simulink model "battery_PV_microgrid"  (R2014a)
settings: Solver=ode23tb  StartTime=0.0  StopTime=86000  MaxStep=0.2  RelTol=1e-5
InitFcn:
  | % Load Stateflow/Controller Parameters
  | controlParams();
  | 
  | % Load Initial Conditions for Model
  | initialConditions();
  | 
  | % Load Battery/PV Parameters
  | parameters();
StopFcn:
  | % Plot results
  | %plotSimResults();
values from neighbouring files (symbols this model uses):
  ambientTemp = 20    [initialConditions.m]    (also in initializeBattery.m)
  currentSat = 0.5    [controlParams.m]    (also in initializeBattery.m)
  desiredBusVoltage = 30    [controlParams.m]    (also in initializeBattery.m = 24.45)
  finalVoltage = 30    [controlParams.m]    (also in initializeBattery.m = 26)
  maxChargeRate = 5    [controlParams.m]    (also in initializeBattery.m)
  maxDischargeRate = -5    [controlParams.m]    (also in initializeBattery.m)
  Ncell = 100    [parameters.m]
  T_init = ambientTemp + 273.15    (= 293.15)    [initialConditions.m]    (also in initializeBattery.m)
  tau = 1e-4    (= 0.0001)    [parameters.m]
undefined symbols (not defined in the file or in its folder): hysteresisSOC, Ion, Lithium, maxSOC, minSOC, optTime, powerHysteresis
undefined symbols (not defined in the file): C1_LUT, C2_LUT, Capacity_LUT, cell_Cp_heat, cell_mass, Em_LUT, PVCellIsc, PVCellRs, PVCellVoc, Qe_init, R0_LUT, R1_LUT, R2_LUT, SOC_LUT, Temperature_LUT
libraries: powerlib x49, fl_lib x18, nesl_utility x6, LiBatteryElements_lib x6, simulink x3, simulink_extras x3, electricdrivelib x1
(part 2 of 2)

== system battery_PV_microgrid/Battery//PV Management and Control/Battery Charge//Discharge Controllers/Battery Charge Controller ==
  Controller Mode : Inport
  Measurements : Inport  Port=2
  Action Port : ActionPort  InitializeStates=reset  ActionType=case
  Bus Selector : BusSelector  OutputSignals=bus.BattVoltage,bus.BattCurrent
  Constant Charge Current : Constant  Value=maxChargeRate
  Final Cell Voltage : Constant  Value=finalVoltage
  Multiport Switch : MultiPortSwitch  DataPortOrder=Zero-based contiguous  Inputs=2
  PID Controller : simulink/Continuous/PID Controller  Controller=PID  TimeDomain=Continuous-time  SampleTime=-1  IntegratorMethod=Forward Euler  FilterMethod=Forward Euler  Form=Parallel  P=1  I=1  D=0.1  N=100  InitialConditionSource=internal  InitialConditionForIntegrator=0  InitialConditionForFilter=0  ExternalReset=none  LimitOutput=on  UpperSaturationLimit=1  LowerSaturationLimit=0  LinearizeAsGain=on  AntiWindupMode=back-calculation  Kb=1  TrackingMode=off  Kt=1  PParamMin=[]  PParamMax=[]  IParamMin=[]  IParamMax=[]  DParamMin=[]  DParamMax=[]  NParamMin=[]  NParamMax=[]  KbParamMin=[]  KbParamMax=[]  KtParamMin=[]  KtParamMax=[]  POutMin=[]  POutMax=[]  IOutMin=[]  IOutMax=[]  DOutMin=[]  DOutMax=[]  NOutMin=[]  NOutMax=[]  KbOutMin=[]  KbOutMax=[]  KtOutMin=[]  KtOutMax=[]  IntegratorOutMin=[]  IntegratorOutMax=[]  FilterOutMin=[]  FilterOutMax=[]  SumOutMin=[]  SumOutMax=[]  SumI1OutMin=[]  SumI1OutMax=[]  SumI2OutMin=[]  SumI2OutMax=[]  SumI3OutMin=[]  SumI3OutMax=[]  SumDOutMin=[]  SumDOutMax=[]  SaturationOutMin=[]  SaturationOutMax=[]  IntegratorContinuousStateAttributes=''  IntegratorStateMustResolveToSignalObject=off  IntegratorRTWStateStorageClass=Auto  FilterContinuousStateAttributes=''  FilterStateMustResolveToSignalObject=off  FilterRTWStateStorageClass=Auto
  Selected Mode : Scope
      settings: ShowLegends=on  TimeRange=4000  YMin=-100  YMax=1400  SaveName=mode
  Sum : Sum  Inputs=|+-
  Sum1 : Sum  Inputs=|+-
  scaling : Subsystem
  Duty : Outport
  wires:
  Multiport Switch/1 -> PID Controller/1
  Constant Charge Current/1 -> Sum/1
  Final Cell Voltage/1 -> Sum1/1
  Sum1/1 -> Multiport Switch/2
  Sum/1 -> Multiport Switch/3
  scaling/1(m) -> Duty/1
  PID Controller/1 -> scaling/1(D)
  Controller Mode/1 -> Selected Mode/1, Multiport Switch/1
  Measurements/1 -> Bus Selector/1
  Bus Selector/1 -> Sum1/2  "<BattVoltage>"
  Bus Selector/2 -> Sum/2  "<BattCurrent>"

== system battery_PV_microgrid/Battery//PV Management and Control/Battery Charge//Discharge Controllers/Battery Discharge Controller ==
  Controller Mode : Inport
  Measurements : Inport  Port=2
  Action Port : ActionPort  InitializeStates=reset  ActionType=default
  Bus Selector : BusSelector  OutputSignals=bus.BattCurrent,bus.BusVoltage
  Maximum Desired Current Output : Constant  Value=maxDischargeRate
  Maximum Desired Current Output1 : Constant  Value=desiredBusVoltage
  Multiport Switch : MultiPortSwitch  DataPortOrder=Zero-based contiguous  Inputs=2
  PID Controller : simulink/Continuous/PID Controller  Controller=PID  TimeDomain=Continuous-time  SampleTime=-1  IntegratorMethod=Forward Euler  FilterMethod=Forward Euler  Form=Parallel  P=1  I=10  D=0  N=100  InitialConditionSource=internal  InitialConditionForIntegrator=0  InitialConditionForFilter=0  ExternalReset=none  LimitOutput=on  UpperSaturationLimit=1  LowerSaturationLimit=0  LinearizeAsGain=on  AntiWindupMode=back-calculation  Kb=1  TrackingMode=off  Kt=1  PParamMin=[]  PParamMax=[]  IParamMin=[]  IParamMax=[]  DParamMin=[]  DParamMax=[]  NParamMin=[]  NParamMax=[]  KbParamMin=[]  KbParamMax=[]  KtParamMin=[]  KtParamMax=[]  POutMin=[]  POutMax=[]  IOutMin=[]  IOutMax=[]  DOutMin=[]  DOutMax=[]  NOutMin=[]  NOutMax=[]  KbOutMin=[]  KbOutMax=[]  KtOutMin=[]  KtOutMax=[]  IntegratorOutMin=[]  IntegratorOutMax=[]  FilterOutMin=[]  FilterOutMax=[]  SumOutMin=[]  SumOutMax=[]  SumI1OutMin=[]  SumI1OutMax=[]  SumI2OutMin=[]  SumI2OutMax=[]  SumI3OutMin=[]  SumI3OutMax=[]  SumDOutMin=[]  SumDOutMax=[]  SaturationOutMin=[]  SaturationOutMax=[]  IntegratorContinuousStateAttributes=''  IntegratorStateMustResolveToSignalObject=off  IntegratorRTWStateStorageClass=Auto  FilterContinuousStateAttributes=''  FilterStateMustResolveToSignalObject=off  FilterRTWStateStorageClass=Auto
  Selected Mode : Scope
      settings: YMin=0.95  YMax=1.05  SaveName=mode2
  Selected Mode1 : Scope
      settings: YMin=0.95  YMax=1.05  SaveName=mode1
  Sum : Sum  Inputs=|+-
  Sum1 : Sum  Inputs=|-+
  scaling : Subsystem
  Duty : Outport
  wires:
  scaling/1(m) -> Duty/1
  Maximum Desired Current Output/1 -> Sum1/1
  Bus Selector/1 -> Sum1/2  "<BattCurrent>"
  Multiport Switch/1 -> Selected Mode1/1, PID Controller/1
  PID Controller/1 -> scaling/1(D)
  Sum1/1 -> Multiport Switch/2
  Sum/1 -> Multiport Switch/3
  Bus Selector/2 -> Sum/2  "<BusVoltage>"
  Controller Mode/1 -> Selected Mode/1, Multiport Switch/1
  Measurements/1 -> Bus Selector/1
  Maximum Desired Current Output1/1 -> Sum/1

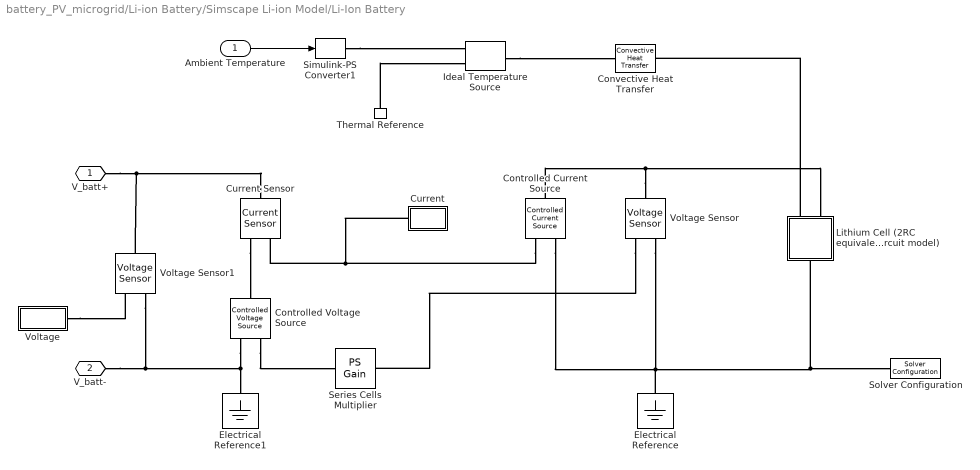
== system battery_PV_microgrid/Li-ion Battery/Simscape Li-ion Model/Li-Ion Battery ==
  Ambient Temperature : Inport
  Controlled Current Source : fl_lib/Electrical/Electrical Sources/Controlled Current Source
  Controlled Voltage Source : fl_lib/Electrical/Electrical Sources/Controlled Voltage Source
  Convective Heat Transfer : fl_lib/Thermal/Thermal Elements/Convective Heat Transfer  area=cell_area m^2  heat_tr_coeff=h_conv W/(m^2 * K)  Q_specify=off  Q_priority=High  Q=0 J/s  T_specify=off  T_priority=High  T=0 K
  Current : Subsystem
  Current Sensor : fl_lib/Electrical/Electrical Sensors/Current Sensor
  Electrical Reference : fl_lib/Electrical/Electrical Elements/Electrical Reference
  Electrical Reference1 : fl_lib/Electrical/Electrical Elements/Electrical Reference
  Ideal Temperature Source : fl_lib/Thermal/Thermal Sources/Ideal Temperature Source
  Lithium Cell (2RC equivalent circuit model) : Subsystem  mask(Lithium battery (two RC-branch equivalent circuit)){Qe_init=Qe_init, T_init=T_init, Capacity_LUT=Capacity_LUT, Em_LUT=Em_LUT, R0_LUT=R0_LUT, R1_LUT=R1_LUT, C1_LUT=C1_LUT, R2_LUT=R2_LUT, C2_LUT=C2_LUT, cell_mass=cell_mass, cell_Cp_heat=cell_Cp_heat, SOC_LUT=SOC_LUT, Temperature_LUT=Temperature_LUT}
      mask prompts: Qe_init "Initial charge deficit (A*hr)"; T_init "Initial cell temperature (K)"; Capacity_LUT "Capacity (A*hr, 1xN table)"; Em_LUT "Em open-circuit voltage (volts, MxN table)"; R0_LUT "R0 terminal resistance (ohms, MxN table)"; R1_LUT "R1 resistance (ohms, MxN table)"; C1_LUT "C1 capacitance (farads, MxN table)"; R2_LUT "R2 resistance (ohms, MxN table)"; C2_LUT "C2 capacitance (farads, MxN table)"; cell_mass "Cell mass (kg)"; cell_Cp_heat "Cell specific heat (J/kg/K)"; SOC_LUT "SOC table breakpoints (Mx1 array)"; Temperature_LUT "Temperature table breakpoints(K, 1xN array)"
      mask Display:
      | image(imread('battery.jpg'))
      | color('red')
      | port_label('LConn',1,'H')
      | port_label('LConn',2,'+')
      | port_label('RConn',1,'-')
  Series Cells Multiplier : fl_lib/Physical Signals/Functions/PS Gain  gain=7
  Simulink-PS Converter1 : nesl_utility/Simulink-PS Converter  PhysicalDomain=network_engine_domain  SubClassName=ps_input  LeftPortType=input  RightPortType=output  PseudoPeriodic=off  Frequencies=[]  NoiseDistribution=none  NoiseParameters=[]  Unit=C  AffineConversion=on  InputFiltering=off  SimscapeFilterOrder=1  InputFilterTimeConstant=.001  UdotUserProvided=1
  Solver Configuration : nesl_utility/Solver Configuration  PhysicalDomain=network_engine_domain  SubClassName=solver  LeftPortType=input  RightPortType=generic  Accelerate=off  Tones=[]  Harmonics=[]  SimulateNoise=off  Profile=off  UseLocalSampling=off  EnableSwitchedLinearOptims=on  FrequencyDomain=off  UseCCode=off  RelTol=0.001  AbsTol=1e-06  MinStep=1e-09  ToWorkspace=off  DoDC=on  ResidualTolerance=1e-9  UseLocalSolver=off  LocalSolverChoice=NE_BACKWARD_EULER_ADVANCER  LocalSolverSampleTime=1  DoFixedCost=off  MaxNonlinIter=3  MaxModeIter=2  LinearAlgebra=Sparse  DelaysMemoryBudget=1024  AutomaticFiltering=on  FilteringTimeConstant=0.001
  Thermal Reference : fl_lib/Thermal/Thermal Elements/Thermal Reference
  Voltage : Subsystem
  Voltage Sensor : fl_lib/Electrical/Electrical Sensors/Voltage Sensor
  Voltage Sensor1 : fl_lib/Electrical/Electrical Sensors/Voltage Sensor
  V_batt+ : PMIOPort  Port=1  Side=Left
  V_batt- : PMIOPort  Port=2  Side=Left
  wires:
  Ambient Temperature/1 -> Simulink-PS Converter1/1
  connections:
  V_batt+/RConn1 -- Voltage Sensor1/LConn1 -- Current Sensor/LConn1
  Controlled Voltage Source/RConn2 -- Voltage Sensor1/RConn2 -- V_batt-/RConn1 -- Electrical Reference1/LConn1
  Lithium Cell (2RC equivalent circuit model)/LConn1 -- Convective Heat Transfer/RConn1
  Thermal Reference/LConn1 -- Ideal Temperature Source/RConn2
  Simulink-PS Converter1/RConn1 -- Ideal Temperature Source/RConn1
  Ideal Temperature Source/LConn1 -- Convective Heat Transfer/LConn1
  Electrical Reference/LConn1 -- Lithium Cell (2RC equivalent circuit model)/RConn1 -- Solver Configuration/RConn1 -- Controlled Current Source/RConn2 -- Voltage Sensor/RConn2
  Controlled Current Source/RConn1 -- Current Sensor/RConn1 -- Current/RConn1
  Controlled Voltage Source/RConn1 -- Series Cells Multiplier/RConn1
  Voltage Sensor/LConn1 -- Lithium Cell (2RC equivalent circuit model)/LConn2 -- Controlled Current Source/LConn1
  Current Sensor/RConn2 -- Controlled Voltage Source/LConn1
  Voltage Sensor/RConn1 -- Series Cells Multiplier/LConn1
  Voltage/RConn1 -- Voltage Sensor1/RConn1

== system battery_PV_microgrid/PV//Battery Power Converters/Buck Converter/scaling ==
  note: Shifting from ]0 to 1[ to a ]-1 to 1[ scale
  D : Inport
  Bias : Bias  Bias=-0.5
  Gain : Gain  Gain=2
  Saturation : Saturate  UpperLimit=1  LowerLimit=-1
  m : Outport
  wires:
  Bias/1 -> Gain/1
  D/1 -> Bias/1
  Gain/1 -> Saturation/1
  Saturation/1 -> m/1

== system battery_PV_microgrid/Battery//PV Management and Control/Battery Charge//Discharge Controllers/Battery Charge Controller/scaling ==
  note: Shifting from ]0 to 1[ to a ]-1 to 1[ scale
  D : Inport
  Bias : Bias  Bias=-0.5
  Gain : Gain  Gain=2
  Saturation : Saturate  UpperLimit=1  LowerLimit=-1
  m : Outport
  wires:
  Saturation/1 -> m/1
  Gain/1 -> Saturation/1
  D/1 -> Bias/1
  Bias/1 -> Gain/1

== system battery_PV_microgrid/Battery//PV Management and Control/Battery Charge//Discharge Controllers/Battery Discharge Controller/scaling ==
  note: Shifting from ]0 to 1[ to a ]-1 to 1[ scale
  D : Inport
  Bias : Bias  Bias=-0.5
  Gain : Gain  Gain=-2
  Saturation : Saturate  UpperLimit=1  LowerLimit=-1
  m : Outport
  wires:
  Saturation/1 -> m/1
  Gain/1 -> Saturation/1
  D/1 -> Bias/1
  Bias/1 -> Gain/1

== system battery_PV_microgrid/Li-ion Battery/Simscape Li-ion Model/Li-Ion Battery/Current ==
  PS-Simulink Converter1 : nesl_utility/PS-Simulink Converter  PhysicalDomain=network_engine_domain  SubClassName=ps_output  LeftPortType=input  RightPortType=output  PseudoPeriodic=off  Frequencies=[]  Unit=A  AffineConversion=off
  PS : PMIOPort  Port=1  Side=Right
  tag scope: I_load=global
  wires:
  PS-Simulink Converter1/1 -> [I_load]
  connections:
  PS-Simulink Converter1/LConn1 -- PS/RConn1

== system battery_PV_microgrid/Li-ion Battery/Simscape Li-ion Model/Li-Ion Battery/Lithium Cell (2RC equivalent circuit model) ==
  " SOC " : Subsystem
  C1 : LiBatteryElements_lib/C_table  C_Table=C1_LUT F  SOC_Table=SOC_LUT  Temp_Table=Temperature_LUT K  v0=0 V
  C2 : LiBatteryElements_lib/C_table  C_Table=C2_LUT F  SOC_Table=SOC_LUT  Temp_Table=Temperature_LUT K  v0=0 V
  Em_table : LiBatteryElements_lib/Em_table  C_Table=Capacity_LUT hr*A  Em_Table=Em_LUT V  SOC_Table=SOC_LUT  Temp_Table=Temperature_LUT K  Qinit=Qe_init hr*A
  Power Sum : fl_lib/Physical Signals/Functions/PS Add
  Power Sum1 : fl_lib/Physical Signals/Functions/PS Add
  R0 : LiBatteryElements_lib/R_table  R_Table=R0_LUT Ohm  SOC_Table=SOC_LUT  Temp_Table=Temperature_LUT K
  R1 : LiBatteryElements_lib/R_table  R_Table=R1_LUT Ohm  SOC_Table=SOC_LUT  Temp_Table=Temperature_LUT K
  R2 : LiBatteryElements_lib/R_table  R_Table=R2_LUT Ohm  SOC_Table=SOC_LUT  Temp_Table=Temperature_LUT K
  T : Subsystem
  Thermal Model : Subsystem
  H : PMIOPort  Tag=PMCPort  Port=1  Side=Left
  + : PMIOPort  Tag=PMCPort  Port=2  Side=Left
  - : PMIOPort  Tag=PMCPort  Port=3  Side=Right
  connections:
  Thermal Model/LConn2 -- H/RConn1
  Em_table/RConn1 -- -/RConn1
  +/RConn1 -- R0/RConn1
  Em_table/LConn1 -- R1/LConn1 -- C1/LConn1
  T/LConn1 -- Thermal Model/RConn1 -- R0/LConn2 -- Em_table/RConn2 -- C1/LConn2 -- R1/LConn2 -- C2/LConn2 -- R2/LConn2
  Power Sum/RConn1 -- Thermal Model/LConn1
  R1/RConn1 -- R2/LConn1 -- C2/LConn1 -- C1/RConn1
  R0/RConn2 -- Power Sum/LConn1
  Power Sum1/RConn1 -- Power Sum/LConn2
  C2/RConn1 -- R0/LConn1 -- R2/RConn1
  Power Sum1/LConn1 -- R2/RConn2
  R1/LConn3 -- C1/LConn3 -- " SOC "/LConn1 -- R0/LConn3 -- C2/LConn3 -- R2/LConn3 -- Em_table/LConn3
  Power Sum1/LConn2 -- R1/RConn2

== system battery_PV_microgrid/Li-ion Battery/Simscape Li-ion Model/Li-Ion Battery/Voltage ==
  PS-Simulink Converter : nesl_utility/PS-Simulink Converter  PhysicalDomain=network_engine_domain  SubClassName=ps_output  LeftPortType=input  RightPortType=output  PseudoPeriodic=off  Frequencies=[]  Unit=V  AffineConversion=off
  PS : PMIOPort  Port=1  Side=Right
  tag scope: V_load=global
  wires:
  PS-Simulink Converter/1 -> [V_load]
  connections:
  PS-Simulink Converter/LConn1 -- PS/RConn1

== system battery_PV_microgrid/Li-ion Battery/Simscape Li-ion Model/Li-Ion Battery/Lithium Cell (2RC equivalent circuit model)/ SOC  ==
  PS-Simulink Converter1 : nesl_utility/PS-Simulink Converter  PhysicalDomain=network_engine_domain  SubClassName=ps_output  LeftPortType=input  RightPortType=output  PseudoPeriodic=off  Frequencies=[]  Unit=1  AffineConversion=off
  PS : PMIOPort  Port=1  Side=Left
  tag scope: SOC=global
  wires:
  PS-Simulink Converter1/1 -> [SOC]
  connections:
  PS/RConn1 -- PS-Simulink Converter1/LConn1

== system battery_PV_microgrid/Li-ion Battery/Simscape Li-ion Model/Li-Ion Battery/Lithium Cell (2RC equivalent circuit model)/T ==
  PS-Simulink Converter1 : nesl_utility/PS-Simulink Converter  PhysicalDomain=network_engine_domain  SubClassName=ps_output  LeftPortType=input  RightPortType=output  PseudoPeriodic=off  Frequencies=[]  Unit=C  AffineConversion=on
  PS : PMIOPort  Port=1  Side=Left
  tag scope: T=global
  wires:
  PS-Simulink Converter1/1 -> [T]
  connections:
  PS/RConn1 -- PS-Simulink Converter1/LConn1

== system battery_PV_microgrid/Li-ion Battery/Simscape Li-ion Model/Li-Ion Battery/Lithium Cell (2RC equivalent circuit model)/Thermal Model ==
  Battery thermal mass : fl_lib/Thermal/Thermal Elements/Thermal Mass  mass=cell_mass kg  sp_heat=cell_Cp_heat J/kg/K  Q_specify=off  Q_priority=High  Q=0 J/s  T_specify=on  T_priority=High  T=T_init K
  Ideal Temperature Sensor : fl_lib/Thermal/Thermal Sensors/Ideal Temperature Sensor
  Ideal Heat Flow Source : fl_lib/Thermal/Thermal Sources/Ideal Heat Flow Source
  Thermal Reference1 : fl_lib/Thermal/Thermal Elements/Thermal Reference
  Thermal Reference2 : fl_lib/Thermal/Thermal Elements/Thermal Reference
  P_in : PMIOPort  Tag=PMCPort  Port=1  Side=Left
  H : PMIOPort  Tag=PMCPort  Port=2  Side=Left
  T : PMIOPort  Tag=PMCPort  Port=3  Side=Right
  connections:
  Thermal Reference2/LConn1 -- Ideal Temperature Sensor/RConn1
  Ideal Temperature Sensor/RConn2 -- T/RConn1
  Thermal Reference1/LConn1 -- Ideal Heat Flow Source/RConn2
  Ideal Temperature Sensor/LConn1 -- H/RConn1 -- Battery thermal mass/LConn1 -- Ideal Heat Flow Source/LConn1
  Ideal Heat Flow Source/RConn1 -- P_in/RConn1

== matlab function battery_PV_microgrid/Battery//PV Management and Control/Optimization Routine/MATLAB Function ==
  data: u input; y output
function y = fcn(u)
%#codegen

% Declare function (contains linprog) as extrinsic
coder.extrinsic('battSolarOptimize');

% Optimizaton parameters
FinalWeight = 50000;    % Weight on the amount of final energy stored

% Battery parameters
Vnominal = 25;  % Nominal terminal voltage [V]
Qnominal = 4;   % Nominal charge [A-h]
pvEff = 0.7;    % Irradiance to Power factor

y = u;

== stateflow chart battery_PV_microgrid/Battery//PV Management and Control/Battery Mode Selection ==
  state storageLogic [parallel]
    settings: executionOrder=1
    state initializeMode
      during:
      batteryMode = 1;
      controlOnOff = 0;
      controlSelect = 0;
    state heuristicLogic
      state disableMode
        during:
        batteryMode = 1;
        controlOnOff = 0;
        controlSelect = 0;
      state dischargeMode
        entry:
        batteryDisengage = 0;
        during:
        batteryMode = 0;
        controlOnOff = 1;
        state constantVoltage
          during:
          controlSelect = 1;
          batteryDisengage = 0;
        state constantCurrent
          during:
          controlSelect = 0;
          batteryDisengage = 0;
        (default) -> storageLogic.heuristicLogic.dischargeMode.constantVoltage : {dischargeHysteresis = 1e-1;}
        storageLogic.heuristicLogic.dischargeMode.constantVoltage -> storageLogic.heuristicLogic.dischargeMode.constantCurrent [order 2] : [gridOnOff == 1]
        storageLogic.heuristicLogic.dischargeMode.constantVoltage -> storageLogic.heuristicLogic.dischargeMode.constantCurrent [order 1] : [measures.Bus.BattCurrent <= maxDischargeRate && after(1,sec)]
        storageLogic.heuristicLogic.dischargeMode.constantCurrent -> storageLogic.heuristicLogic.dischargeMode.constantVoltage : [(measures.Bus.BattCurrent > maxDischargeRate + dischargeHysteresis || ...
            | measures.Bus.BusVoltage > desiredBusVoltage + dischargeHysteresis) && (after(1,sec) && gridOnOff == 0) ]
      state chargeMode
        during:
        batteryMode = 1;
        controlOnOff = 1;
        state constantVoltage
          during:
          controlSelect = 0;
          batteryDisengage = 0;
        state constantCurrent
          during:
          controlSelect = 1;
          batteryDisengage = 0;
        state currentSaturate
          during:
          controlSelect = 0;
          batteryDisengage = 1;
        (default) -> storageLogic.heuristicLogic.chargeMode.constantCurrent : {chargeHysteresis = 0.1;}
        storageLogic.heuristicLogic.chargeMode.constantCurrent -> storageLogic.heuristicLogic.chargeMode.constantVoltage : [finalVoltage <= measures.Bus.BattVoltage  && ...
            | after(1, sec)]
        storageLogic.heuristicLogic.chargeMode.constantVoltage -> storageLogic.heuristicLogic.chargeMode.currentSaturate [order 2] : [measures.Bus.BattCurrent <= currentSat]
        storageLogic.heuristicLogic.chargeMode.constantVoltage -> storageLogic.heuristicLogic.chargeMode.constantCurrent [order 1] : [finalVoltage > measures.Bus.BattVoltage + chargeHysteresis && ...
            | after(1, sec) ]
      (junction 153) -> (junction 148) [order 2] : % Battery cannot be charged
          | [measures.Battery.SOC < maxSOC - hysteresisSOC]
      (junction 153) -> (junction 145) [order 1] : % Battery cannot be fully discharged
          | [measures.Battery.SOC > minSOC + hysteresisSOC]
      (junction 148) -> storageLogic.heuristicLogic.chargeMode : % Charge mode to store excess PV
          | [measures.PV.Power > measures.Load.Power]
      storageLogic.heuristicLogic.disableMode -> (junction 153) : % Battery must be enabled
          | [switches.battery == 1]
      (junction 145) -> storageLogic.heuristicLogic.dischargeMode : % Dischage mode to supply PV difference
          | [measures.PV.Power < measures.Load.Power]
      storageLogic.heuristicLogic.dischargeMode -> storageLogic.heuristicLogic.disableMode [order 1] : % Manual shutdown of battery
          | [switches.battery == 0]
      storageLogic.heuristicLogic.chargeMode -> storageLogic.heuristicLogic.disableMode [order 1] : % Manual shutdown of battery
          | [switches.battery == 0]
      storageLogic.heuristicLogic.chargeMode -> storageLogic.heuristicLogic.disableMode [order 2] : % Battery fully charged
          | [measures.Battery.SOC > maxSOC]
      storageLogic.heuristicLogic.dischargeMode -> storageLogic.heuristicLogic.disableMode [order 2] : % Battery fully discharged
          | [measures.Battery.SOC < minSOC]
      storageLogic.heuristicLogic.chargeMode -> (junction 168) [order 3] : % Rate limit switching
          | [after(5,sec)]
      (junction 171) -> storageLogic.heuristicLogic.chargeMode
      storageLogic.heuristicLogic.dischargeMode -> (junction 165) [order 3] : % Rate limit switching
          | [after(5,sec)]
      (junction 169) -> storageLogic.heuristicLogic.dischargeMode
      (default) -> storageLogic.heuristicLogic.disableMode
      (junction 165) -> (junction 171) : % Charge mode to store excess PV
          | [measures.PV.Power > measures.Load.Power]
      (junction 168) -> (junction 169) : % Dischage mode to supply PV difference
          | [measures.PV.Power < measures.Load.Power]
    state optimizationLogic
      state disableMode
        during:
        batteryMode = 1;
        controlOnOff = 0;
        controlSelect = 0;
      state dischargeMode
        entry:
        batteryDisengage = 0;
        during:
        batteryMode = 0;
        controlOnOff = 1;
        state constantVoltage
          during:
          controlSelect = 1;
          batteryDisengage = 0;
        state constantCurrent
          during:
          controlSelect = 0;
          batteryDisengage = 0;
        (default) -> storageLogic.optimizationLogic.dischargeMode.constantVoltage : {dischargeHysteresis = 1e-1;}
        storageLogic.optimizationLogic.dischargeMode.constantVoltage -> storageLogic.optimizationLogic.dischargeMode.constantCurrent [order 2] : [gridOnOff == 1]
        storageLogic.optimizationLogic.dischargeMode.constantVoltage -> storageLogic.optimizationLogic.dischargeMode.constantCurrent [order 1] : [measures.Bus.BattCurrent <= maxDischargeRate && after(1,sec)]
        storageLogic.optimizationLogic.dischargeMode.constantCurrent -> storageLogic.optimizationLogic.dischargeMode.constantVoltage : [(measures.Bus.BattCurrent > maxDischargeRate + dischargeHysteresis || ...
            | measures.Bus.BusVoltage > desiredBusVoltage + dischargeHysteresis) && (after(1,sec) && gridOnOff == 0) ]
      state chargeMode
        during:
        batteryMode = 1;
        controlOnOff = 1;
        state constantVoltage
          during:
          controlSelect = 0;
          batteryDisengage = 0;
        state constantCurrent
          during:
          controlSelect = 1;
          batteryDisengage = 0;
        state currentSaturate
          during:
          controlSelect = 0;
          batteryDisengage = 1;
        (default) -> storageLogic.optimizationLogic.chargeMode.constantCurrent : {chargeHysteresis = 0.1;}
        storageLogic.optimizationLogic.chargeMode.constantCurrent -> storageLogic.optimizationLogic.chargeMode.constantVoltage : [finalVoltage <= measures.Bus.BattVoltage  && ...
            | after(1, sec)]
        storageLogic.optimizationLogic.chargeMode.constantVoltage -> storageLogic.optimizationLogic.chargeMode.currentSaturate [order 2] : [measures.Bus.BattCurrent <= currentSat]
        storageLogic.optimizationLogic.chargeMode.constantVoltage -> storageLogic.optimizationLogic.chargeMode.constantCurrent [order 1] : [finalVoltage > measures.Bus.BattVoltage + chargeHysteresis && ...
            | after(1, sec) ]
      (junction 191) -> (junction 190) [order 2] : % Battery cannot be charged
          | [measures.Battery.SOC < maxSOC - hysteresisSOC]
      (junction 191) -> (junction 192) [order 1] : % Battery cannot be fully discharged
          | [measures.Battery.SOC > minSOC + hysteresisSOC]
      (junction 190) -> storageLogic.optimizationLogic.chargeMode : % Charge mode to store excess PV
          | [measures.PV.Power > measures.Load.Power]
      storageLogic.optimizationLogic.disableMode -> (junction 191) : % Battery must be enabled
          | [switches.battery == 1]
      (junction 192) -> storageLogic.optimizationLogic.dischargeMode : % Dischage mode to supply PV difference
          | [measures.PV.Power < measures.Load.Power]
      storageLogic.optimizationLogic.dischargeMode -> storageLogic.optimizationLogic.disableMode [order 1] : % Manual shutdown of battery
          | [switches.battery == 0]
      storageLogic.optimizationLogic.chargeMode -> storageLogic.optimizationLogic.disableMode [order 1] : % Manual shutdown of battery
          | [switches.battery == 0]
      storageLogic.optimizationLogic.chargeMode -> storageLogic.optimizationLogic.disableMode [order 2] : % Battery fully charged
          | [measures.Battery.SOC > maxSOC]
      storageLogic.optimizationLogic.dischargeMode -> storageLogic.optimizationLogic.disableMode [order 2] : % Battery fully discharged
          | [measures.Battery.SOC < minSOC]
      storageLogic.optimizationLogic.chargeMode -> (junction 195) [order 3] : % Rate limit switching
          | [after(5,sec)]
      (junction 193) -> storageLogic.optimizationLogic.chargeMode
      storageLogic.optimizationLogic.dischargeMode -> (junction 194) [order 3] : % Rate limit switching
          | [after(5,sec)]
      (junction 196) -> storageLogic.optimizationLogic.dischargeMode
      (default) -> storageLogic.optimizationLogic.disableMode
      (junction 194) -> (junction 193) : % Charge mode to store excess PV
          | [measures.PV.Power > measures.Load.Power]
      (junction 195) -> (junction 196) : % Dischage mode to supply PV difference
          | [measures.PV.Power < measures.Load.Power]
    (default) -> initializeMode
    initializeMode -> heuristicLogic : % Allow for system transients
        | [after(10,sec)]
    heuristicLogic -> optimizationLogic : [switches.opt == 1]
    optimizationLogic -> heuristicLogic : [switches.opt ~= 1]
  state gridLogic [parallel]
    during:
    maxPower = finalVoltage*(maxChargeRate - 1);
    minPower = -finalVoltage*(maxDischargeRate + 1);
    settings: executionOrder=2
    state disconnectGrid
      during:
      gridOnOff = 0;
    state connectGrid
      during:
      gridOnOff = 1;
    (junction 120) -> (junction 122) [order 1] : % Connect grid to absorb excess PV
        | [measures.PV.Power - measures.Load.Power > maxPower + powerHysteresis]
    (junction 120) -> (junction 122) [order 2] : % Connect grid to supply beyond battery
        | [measures.Load.Power - measures.PV.Power > minPower - 2*powerHysteresis]
    (junction 113) -> (junction 120) [order 2] : % Battery is enabled
        | [controlOnOff == 1]
    (junction 122) -> (junction 117) : % Prevent bus chatter
        | [measures.Grid.Power < measures.Load.Power]
    (junction 117) -> connectGrid
    (junction 113) -> (junction 117) [order 1] : % Battery manually disabled
        | [controlOnOff == 0]
    disconnectGrid -> (junction 113)
    (default) -> connectGrid
    connectGrid -> (junction 126)
    (junction 126) -> (junction 131) [order 1] : % Disable grid since PV supplies all power
        | [measures.PV.Power - measures.Load.Power < maxPower]
    (junction 131) -> (junction 132) : % Disable grid since battery can supply all power
        | [(measures.Load.Power - measures.PV.Power < minPower + powerHysteresis) && after(1,sec)]
    (junction 132) -> disconnectGrid : % Battery is enabled
        | [controlOnOff == 1]
    (junction 126) -> (junction 137) [order 2] : [measures.Bus.BattPower > 0]
    (junction 137) -> (junction 132) : [measures.PV.Power < measures.Load.Power]
  data: controlOnOff output; switches input; batteryMode output; batteryDisengage local; chargeHysteresis local; dischargeHysteresis local; currentSat parameter; finalVoltage parameter; controlSelect output; maxDischargeRate parameter; desiredBusVoltage parameter; measures input Bus: Measurements; gridOnOff output; maxSOC parameter; minSOC parameter; hysteresisSOC parameter; powerHysteresis parameter; maxChargeRate parameter; maxPower local; minPower local
